simulink model "mvdc_mpc"  (R2018b)
settings: configuration reference "Active" (kept outside this file)
undefined symbols (not defined in the file): A_VehicleReference_m2, acc_control_learning, ax_lim_mps2, ay_lim_mps2, DiscIntNeverNeededParam, drag_coefficient, l_front_m, l_rear_m, LatAcc_cov_debug, LatAcc_FFweights, LatAcc_mean_debug, LongAcc_FFweights, P_VDC_axFFModelLearningEnable, P_VDC_axFFModelLearningRate, P_VDC_axFFModelLearningReg, P_VDC_ayFFModelLearningEnable, P_VDC_ayFFModelLearningRate, P_VDC_ayFFModelLearningReg, P_VDC_Dist_ax_perc, P_VDC_Dist_ay_perc, P_VDC_EnableNumLatErrorDer_b, P_VDC_EnableTubeMPC, P_VDC_EnableUncertaintyLearning, P_VDC_EnableYawRateAccRepl, P_VDC_LatAcc_BetaGain, P_VDC_LatAcc_EnableForesightFF, P_VDC_LatAcc_FF_Ts, P_VDC_LatAcc_Steering_Ts, P_VDC_LatAcc_UndersteerComp_Ts, P_VDC_LatAcc_VehicleDynamics_Ts, P_VDC_LatAccKi, P_VDC_LatAccKi_Lim_perc, P_VDC_LatAccKp_ay, P_VDC_LatAccKp_Delta, P_VDC_LatErrorDer_Ts_s, P_VDC_LongAcc_EnableForesightFF, P_VDC_LongAcc_FB_Ts, P_VDC_LongAcc_FF_Ts, P_VDC_LongAcc_LimFb_N, P_VDC_LongAccKp, P_VDC_MaxTightening, P_VDC_MinVelSlipCalc_mps, P_VDC_PositiveAxLimScale, P_VDC_StabilizerRearSideSlip_rad, P_VDC_SteeringOvalComp_rad, P_VDC_SteeringSteadyStateUndersteerComp_rad, P_VDC_UncertaintyLearningGain, P_VDC_UncertaintyLearningSamples, P_VDC_UncertaintyTarget_perc, P_VDC_VirtualController, Pos, roh_air, sys, tS, tSSlow, TUMHealthStatus, v_mps, vehiclemass_kg
libraries: simulink x31
(part 1 of 2)
settings Model: DataDictionary=mvdc_mpc.sldd  PauseTimes=19.88  Creator=wischnewski  LastModifiedBy=ge34qer

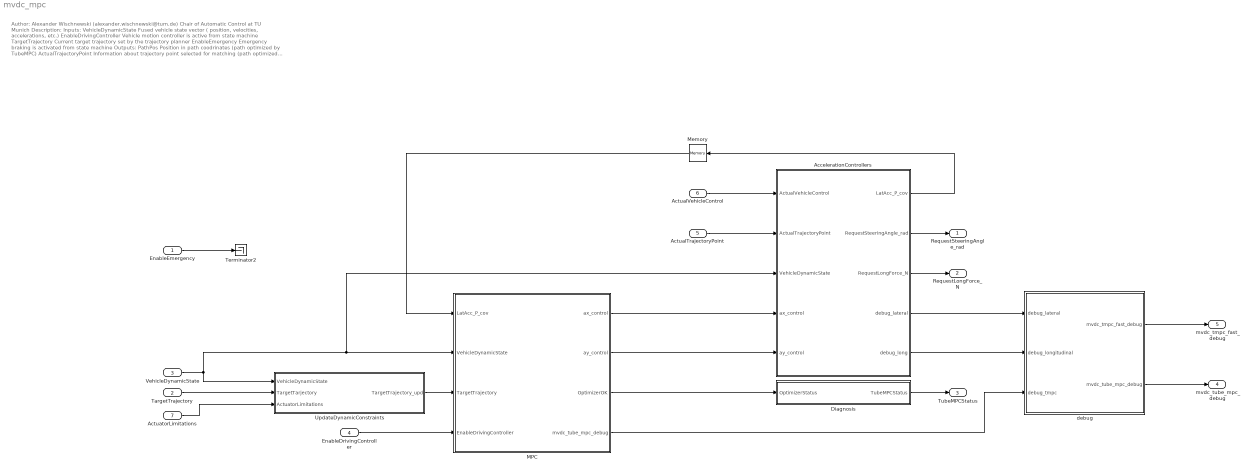
== system mvdc_mpc ==
  note: Author: Alexander Wischnewski (alexander.wischnewski@tum.de)
      | Chair of Automatic Control at TU Munich
      |
      | Description:
      |
      | Inputs:
      | VehicleDynamicState Fused vehicle state vector ( position, velocities, accelerations, etc.)
      | EnableDrivingController Vehicle motion controller is active from state machine
      | TargetTrajectory Current target trajectory set by the trajectory planner
      | EnableEmergency Emergency braking is activated from state machine
      |
      | Outputs:
      | PathPos Position in path coodrinates (path optimized by TubeMPC)
      | ActualTrajectoryPoint Information about trajectory point selected for matching (path optimized by TubeMPC)
      | OptimizedTrajectory Trajectory optimized by TubeMPC
      | TubeMPCStatus Status of TubeMPC controller
  EnableEmergency : Inport  OutDataTypeStr=boolean
  TargetTrajectory : Inport  Port=2  OutDataTypeStr=Bus: Trajectory  SampleTime=tS  BusOutputAsStruct=on
  VehicleDynamicState : Inport  Port=3  OutDataTypeStr=Bus: VehicleDynamicState  SampleTime=tS
  EnableDrivingController : Inport  Port=4  OutDataTypeStr=boolean  SampleTime=tS
  ActualTrajectoryPoint : Inport  Port=5  OutDataTypeStr=Bus: TrajectoryPoint  PortDimensions=1  BusOutputAsStruct=on
  ActualVehicleControl : Inport  Port=6  OutDataTypeStr=Bus: VehicleControl
  ActuatorLimitations : Inport  Port=7  OutDataTypeStr=Bus: ActuatorLimitations  BusOutputAsStruct=on
  AccelerationControllers : Subsystem
  Diagnosis : Subsystem
  MPC : Subsystem
  Memory : Memory
  Terminator2 : Terminator
  UpdateDynamicConstraints : Subsystem
  debug : Subsystem
  RequestSteeringAngle_rad : Outport  SampleTime=tS
  RequestLongForce_N : Outport  Port=2  SampleTime=tS
  TubeMPCStatus : Outport  Port=3  OutDataTypeStr=Enum: TUMHealthStatus  SampleTime=tS
  mvdc_tube_mpc_debug : Outport  Port=4  OutDataTypeStr=Bus: mvdc_tube_mpc_debug  SampleTime=tS
  mvdc_tmpc_fast_debug : Outport  Port=5  OutDataTypeStr=Bus: mvdc_tmpc_fast_debug  SampleTime=tS
  wires:
  UpdateDynamicConstraints/1(TargetTrajectory_upd) -> MPC/3(TargetTrajectory)
  VehicleDynamicState/1 -> MPC/2(VehicleDynamicState), AccelerationControllers/3(VehicleDynamicState), UpdateDynamicConstraints/1(VehicleDynamicState)
  Diagnosis/1(TubeMPCStatus) -> TubeMPCStatus/1
  MPC/3(OptimizerOK) -> Diagnosis/1(OptimizerStatus)
  EnableEmergency/1 -> Terminator2/1
  AccelerationControllers/2(RequestSteeringAngle_rad) -> RequestSteeringAngle_rad/1
  AccelerationControllers/3(RequestLongForce_N) -> RequestLongForce_N/1
  MPC/1(ax_control) -> AccelerationControllers/4(ax_control)
  MPC/2(ay_control) -> AccelerationControllers/5(ay_control)
  AccelerationControllers/4(debug_lateral) -> debug/1(debug_lateral)
  AccelerationControllers/5(debug_long) -> debug/2(debug_longitudinal)
  MPC/4(mvdc_tube_mpc_debug) -> debug/3(debug_tmpc)
  ActualVehicleControl/1 -> AccelerationControllers/1(ActualVehicleControl)
  debug/1(mvdc_tmpc_fast_debug) -> mvdc_tmpc_fast_debug/1
  debug/2(mvdc_tube_mpc_debug) -> mvdc_tube_mpc_debug/1
  ActualTrajectoryPoint/1 -> AccelerationControllers/2(ActualTrajectoryPoint)
  ActuatorLimitations/1 -> UpdateDynamicConstraints/3(ActuatorLimitations)
  TargetTrajectory/1 -> UpdateDynamicConstraints/2(TargetTarjectory)
  Memory/1 -> MPC/1(LatAcc_P_cov)
  AccelerationControllers/1(LatAcc_P_cov) -> Memory/1
  EnableDrivingController/1 -> MPC/4(EnableDrivingController)

== system mvdc_mpc/AccelerationControllers ==
  note: These controllers add small correction signal to the requested steering angle
      | and longitudinal force to counteract small uncertainties in the request characteristics.
      |
      | They do not interfer with the constraint satisfaction generated by the TMPC controller
      | as it is assumed that the measured accelerations are correct and therefore the controller
      | only compensates errors in the request characteristic.
  ActualVehicleControl : Inport
  ActualTrajectoryPoint : Inport  Port=2  OutDataTypeStr=Bus: TrajectoryPoint  PortDimensions=1  BusOutputAsStruct=on
  VehicleDynamicState : Inport  Port=3
  ax_control : Inport  Port=4
  ay_control : Inport  Port=5
  LateralController : Subsystem
  LongitudinalController : Subsystem
  Terminator : Terminator
  LatAcc_P_cov : Outport
  RequestSteeringAngle_rad : Outport  Port=2  SampleTime=tS
  RequestLongForce_N : Outport  Port=3  SampleTime=tS
  debug_lateral : Outport  Port=4
  debug_long : Outport  Port=5
  wires:
  VehicleDynamicState/1 -> LongitudinalController/2(VehicleDynamicState), LateralController/1(VehicleDynamicState)
  ay_control/1 -> LateralController/2(Target_ay_mps2)
  LateralController/1(RequestSteeringAngle_rad) -> RequestSteeringAngle_rad/1
  ax_control/1 -> LongitudinalController/3(Target_ax_mps2)
  LongitudinalController/1(RequestLongForce_N) -> RequestLongForce_N/1
  LateralController/2(debug) -> debug_lateral/1
  LongitudinalController/2(debug) -> debug_long/1
  ActualVehicleControl/1 -> Terminator/1
  ActualTrajectoryPoint/1 -> LateralController/3(ActualTrajectoryPoint)
  LateralController/3(LatAcc_P_cov) -> LatAcc_P_cov/1
  LateralController/4(StabilizerActive) -> LongitudinalController/1(StabilizerActive)

== system mvdc_mpc/Diagnosis ==
  OptimizerStatus : Inport
  Constant : Constant  Value=TUMHealthStatus.OK
  Constant1 : Constant  Value=TUMHealthStatus.ERROR
  Switch : Switch  Criteria=u2 > Threshold
  TubeMPCStatus : Outport
  wires:
  Switch/1 -> TubeMPCStatus/1
  OptimizerStatus/1 -> Switch/2
  Constant/1 -> Switch/1
  Constant1/1 -> Switch/3

== system mvdc_mpc/MPC ==
  LatAcc_P_cov : Inport
  VehicleDynamicState : Inport  Port=2  OutDataTypeStr=Bus: VehicleDynamicState
  TargetTrajectory : Inport  Port=3  OutDataTypeStr=Bus: Trajectory
  EnableDrivingController : Inport  Port=4  OutDataTypeStr=boolean  SampleTime=tS
  Bus Selector : BusSelector  OutputSignals=ax_pred_mps2,ay_pred_mps2
  Debug : Subsystem
  DelayCompensation : Subsystem
  DisturbanceEstimation : Subsystem
  Memory : Memory  InheritSampleTime=on
  Memory1 : Memory  InheritSampleTime=on
  TubeMPC : Subsystem  TreatAsAtomicUnit=on
  VehicleReadyForTMPC : Subsystem
  ax_control : Outport
  ay_control : Outport  Port=2
  OptimizerOK : Outport  Port=3  OutDataTypeStr=boolean
  mvdc_tube_mpc_debug : Outport  Port=4  OutDataTypeStr=Bus: mvdc_tube_mpc_debug
  wires:
  TargetTrajectory/1 -> VehicleReadyForTMPC/2(TargetTrajectory), TubeMPC/5(TargetTrajectory), Debug/9(TargetTrajectory)
  VehicleDynamicState/1 -> DelayCompensation/1(VehicleDynamicState), DisturbanceEstimation/3(VehicleDynamicState), VehicleReadyForTMPC/1(VehicleDynamicState)
  Debug/1(mvdc_tube_mpc_debug) -> mvdc_tube_mpc_debug/1
  TubeMPC/3(solver_details) -> Debug/4(solver_details)
  TubeMPC/2(exitflags) -> Debug/3(exit_flags)
  TubeMPC/5(MiscDebug) -> Debug/6(MiscDebug)
  TubeMPC/4(ResampledTargetTrajectory) -> Debug/5(ResampledTargetTrajectory)
  TubeMPC/1(OptimizerOK) -> OptimizerOK/1
  TubeMPC/7(Linearization) -> Debug/8(LinearizationDebug)
  DelayCompensation/1(VehicleDynamicStateUpdated) -> TubeMPC/1(VehicleDynamicState), Debug/2(VehicleDynamicState)
  Memory/1 -> DisturbanceEstimation/1(ax_control_mps2)
  Memory1/1 -> DisturbanceEstimation/2(ay_control_mps2)
  DisturbanceEstimation/2(M_tilde) -> TubeMPC/2(M_tilde)
  DisturbanceEstimation/1(debug) -> Debug/1(debug_distLearning)
  TubeMPC/6(Prediction) -> Bus Selector/1, Debug/7(PredictionDebug)
  Bus Selector/1 -> Memory/1, ax_control/1  "<ax_pred_mps2>"
  Bus Selector/2 -> ay_control/1, Memory1/1  "<ay_pred_mps2>"
  LatAcc_P_cov/1 -> TubeMPC/4(LatAcc_P_cov)
  VehicleReadyForTMPC/1(VehicleReadyForTMPC) -> DisturbanceEstimation/4(VehicleReadyForTMPC), TubeMPC/Enable
  EnableDrivingController/1 -> VehicleReadyForTMPC/3(EnableDrivingController)
  VehicleReadyForTMPC/2(StartTMPC) -> TubeMPC/3(StartTMPC)

== system mvdc_mpc/UpdateDynamicConstraints ==
  note: reduce the max. long acceleration at standstill
      | to prevent excessive wheelspin at the start.
  note: calculates the maximum possible lateral acceleration
      | at low speeds and checks whether the steering angle
      | limits the achievable lateral acceleration.
  VehicleDynamicState : Inport  OutDataTypeStr=Bus: VehicleDynamicState  SampleTime=tS
  TargetTarjectory : Inport  Port=2
  ActuatorLimitations : Inport  Port=3  OutDataTypeStr=Bus: ActuatorLimitations  BusOutputAsStruct=on
  Bus Assignment : BusAssignment  AssignedSignals=ax_lim_mps2,ay_lim_mps2
  Bus Selector : BusSelector  OutputSignals=SteeringAngleMax_rad
  Bus Selector1 : BusSelector  OutputSignals=v_mps
  Bus Selector2 : BusSelector  OutputSignals=ay_lim_mps2
  Bus Selector3 : BusSelector  OutputSignals=ax_lim_mps2
  Constant : Constant  Value=P_VDC_MinVelSlipCalc_mps
  Gain : Gain  Gain=1/(l_front_m+l_rear_m)
  Gain1 : Gain  Gain=1/3
  Min : MinMax  Inputs=2
  Min1 : MinMax  Function=max  Inputs=2
  Multiply : Product
  Square : Math  Operator=square  SaturateOnIntegerOverflow=on
  Switch : Switch  Criteria=u2 > Threshold  Threshold=P_VDC_MinVelSlipCalc_mps
  TargetTrajectory_upd : Outport
  wires:
  ActuatorLimitations/1 -> Bus Selector/1
  Bus Selector/1 -> Gain/1  "<SteeringAngleMax_rad>"
  VehicleDynamicState/1 -> Bus Selector1/1
  Square/1 -> Multiply/2
  Gain/1 -> Multiply/1
  Bus Selector2/1 -> Min/1  "<ay_lim_mps2>"
  Min/1 -> Bus Assignment/3
  Bus Assignment/1 -> TargetTrajectory_upd/1
  Bus Selector1/1 -> Switch/2, Min1/1  "<v_mps>"
  Constant/1 -> Min1/2
  Min1/1 -> Square/1
  Multiply/1 -> Min/2
  TargetTarjectory/1 -> Bus Assignment/1, Bus Selector2/1, Bus Selector3/1
  Switch/1 -> Bus Assignment/2
  Bus Selector3/1 -> Gain1/1, Switch/1  "<ax_lim_mps2>"
  Gain1/1 -> Switch/3

== system mvdc_mpc/debug ==
  note: the tmpc_cnt enables sync between different logging rates
  debug_lateral : Inport
  debug_longitudinal : Inport  Port=2
  debug_tmpc : Inport  Port=3
  Bus Assignment : BusAssignment  AssignedSignals=LongAcc_FFweights,LatAcc_FFweights,LatAcc_mean_debug,LatAcc_cov_debug
  Bus Creator : BusCreator  Inputs=39
  Bus Selector : BusSelector  OutputSignals=LatAcc_bank_mps2,LatAcc_FB_Dist_rad,LatAcc_FB_ay_rad,LatAcc_FB_Delta_rad,LatAcc_FFss_rad,LatAcc_FFdyn_rad,LatAcc_Control_rad,LatAcc_Target_mps2,LatAcc_VirtualAccTarget_mps2,LatAcc_VirtualSteeringTarget_rad,LatAcc_FFLearned_rad,LatAcc_DiffToNeutralSteer_rad,LatAcc_FBStabilizer_rad
  Bus Selector1 : BusSelector  OutputSignals=LongAcc_FB_N,LongAcc_FFax_N,LongAcc_FFdist_N,LongAcc_Control_N,LongAcc_Target_mps2,LongAcc_TargetFF_mps2,LongAcc_FFLearned_N
  Bus Selector2 : BusSelector  OutputSignals=cost_values,solver_iteration,solver_state,solver_runTime_s,solver_pri_res,solver_dua_res,tmpc_cnt,TireUtilizationTarget,ax_LearnedBound_mps2,ax_DataCoverage_perc,ax_Uncertainty_mps2,ay_LearnedBound_mps2,ay_DataCoverage_perc,ay_Uncertainty_mps2,dot_d_analytical_mps,dot_d_numerical_mps
  Bus Selector3 : BusSelector  OutputSignals=LatAcc_FFweights,LatAcc_mean_debug,LatAcc_cov_debug
  Bus Selector4 : BusSelector  OutputSignals=LongAcc_FFweights
  Demux : Demux
  Signal Copy{2..5} (4 alike) : SignalConversion  OverrideOpt=off
  mvdc_tmpc_fast_debug : Outport
  mvdc_tube_mpc_debug : Outport  Port=2  OutDataTypeStr=Bus: mvdc_tube_mpc_debug  SampleTime=tS
  wires:
  debug_longitudinal/1 -> Bus Selector4/1, Bus Selector1/1
  Bus Selector1/2 -> Bus Creator/15  "<LongAcc_FFax_N>"
  Bus Selector/5 -> Bus Creator/5  "<LatAcc_FFss_rad>"
  Bus Selector/3 -> Bus Creator/3  "<LatAcc_FB_ay_rad>"
  Bus Selector/7 -> Bus Creator/7  "<LatAcc_Control_rad>"
  Bus Selector1/3 -> Bus Creator/16  "<LongAcc_FFdist_N>"
  Bus Selector1/4 -> Bus Creator/17  "<LongAcc_Control_N>"
  debug_lateral/1 -> Bus Selector3/1, Bus Selector/1
  Bus Selector2/7 -> Bus Creator/30  "<tmpc_cnt>"
  Bus Selector/8 -> Bus Creator/8  "<LatAcc_Target_mps2>"
  Bus Selector1/5 -> Bus Creator/18  "<LongAcc_Target_mps2>"
  Bus Selector2/2 -> Bus Creator/25  "<solver_iteration>"
  Bus Selector2/1 -> Demux/1  "<cost_values>"
  Demux/1 -> Signal Copy2/1
  Demux/2 -> Signal Copy3/1
  Signal Copy3/1 -> Bus Creator/22  "input_cost"
  Demux/3 -> Signal Copy4/1
  Signal Copy4/1 -> Bus Creator/23  "reg_cost"
  Demux/4 -> Signal Copy5/1
  Signal Copy5/1 -> Bus Creator/24  "slack_cost"
  Bus Selector2/4 -> Bus Creator/27  "<solver_runTime_s>"
  Bus Selector2/5 -> Bus Creator/28  "<solver_pri_res>"
  Bus Selector2/6 -> Bus Creator/29  "<solver_dua_res>"
  Bus Creator/1 -> mvdc_tmpc_fast_debug/1
  Bus Selector/11 -> Bus Creator/11  "<LatAcc_FFLearned_rad>"
  Bus Selector1/1 -> Bus Creator/14  "<LongAcc_FB_N>"
  Signal Copy2/1 -> Bus Creator/21  "state_cost"
  Bus Selector2/3 -> Bus Creator/26  "<solver_state>"
  Bus Selector2/8 -> Bus Creator/31  "<TireUtilizationTarget>"
  Bus Selector2/9 -> Bus Creator/32  "<ax_LearnedBound_mps2>"
  Bus Selector2/10 -> Bus Creator/33  "<ax_DataCoverage_perc>"
  Bus Selector2/12 -> Bus Creator/35  "<ay_LearnedBound_mps2>"
  Bus Selector2/13 -> Bus Creator/36  "<ay_DataCoverage_perc>"
  Bus Selector2/11 -> Bus Creator/34  "<ax_Uncertainty_mps2>"
  Bus Selector2/14 -> Bus Creator/37  "<ay_Uncertainty_mps2>"
  Bus Selector1/7 -> Bus Creator/20  "<LongAcc_FFLearned_N>"
  debug_tmpc/1 -> Bus Assignment/1, Bus Selector2/1
  Bus Assignment/1 -> mvdc_tube_mpc_debug/1
  Bus Selector3/1 -> Bus Assignment/3  "<LatAcc_FFweights>"
  Bus Selector4/1 -> Bus Assignment/2  "<LongAcc_FFweights>"
  Bus Selector/9 -> Bus Creator/9  "<LatAcc_VirtualAccTarget_mps2>"
  Bus Selector1/6 -> Bus Creator/19  "<LongAcc_TargetFF_mps2>"
  Bus Selector/6 -> Bus Creator/6  "<LatAcc_FFdyn_rad>"
  Bus Selector/1 -> Bus Creator/1  "<LatAcc_bank_mps2>"
  Bus Selector/4 -> Bus Creator/4  "<LatAcc_FB_Delta_rad>"
  Bus Selector/10 -> Bus Creator/10  "<LatAcc_VirtualSteeringTarget_rad>"
  Bus Selector/2 -> Bus Creator/2  "<LatAcc_FB_Dist_rad>"
  Bus Selector3/2 -> Bus Assignment/4  "<LatAcc_mean_debug>"
  Bus Selector3/3 -> Bus Assignment/5  "<LatAcc_cov_debug>"
  Bus Selector/12 -> Bus Creator/12  "<LatAcc_DiffToNeutralSteer_rad>"
  Bus Selector/13 -> Bus Creator/13  "<LatAcc_FBStabilizer_rad>"
  Bus Selector2/15 -> Bus Creator/38  "<dot_d_analytical_mps>"
  Bus Selector2/16 -> Bus Creator/39  "<dot_d_numerical_mps>"

== system mvdc_mpc/AccelerationControllers/LateralController ==
  note: used to disable throttle in case
      | stabilizer kicks in
  VehicleDynamicState : Inport
  Target_ay_mps2 : Inport  Port=2
  ActualTrajectoryPoint : Inport  Port=3  OutDataTypeStr=Bus: TrajectoryPoint  PortDimensions=1  BusOutputAsStruct=on
  Abs : Abs
  Add : Sum  Inputs=+++++++
  Add1 : Sum  Inputs=++++++
  Bus Creator : BusCreator  Inputs=16
  Bus Selector : BusSelector  OutputSignals=ay_lim_mps2
  Bus Selector1 : BusSelector  OutputSignals=valid_IMU_b,alphaRL_rad,alphaRR_rad,DeltaWheel_rad,dPsi_radps,ay_mps2,v_mps
  Compare To Constant : simulink/Logic and Bit Operations/Compare To Constant  relop=>  const=0  OutDataTypeStr=boolean
  Constant : Constant  Value=0
  Feedback : Subsystem
  Feedforward_InverseModel : Subsystem
  Feedforward_Learning : Subsystem
  Selector : Selector  InputPortWidth=sys.N_hor+1  IndexOptions=Index vector (dialog)  Indices=1  OutputSizes=1
  Unit Delay1 : UnitDelay  SampleTime=-1
  RequestSteeringAngle_rad : Outport
  debug : Outport  Port=2
  LatAcc_P_cov : Outport  Port=3
  StabilizerActive : Outport  Port=4
  wires:
  Target_ay_mps2/1 -> Feedforward_InverseModel/2(LatAcc_Target_mps2), Selector/1
  VehicleDynamicState/1 -> Bus Selector1/1
  Add/1 -> Bus Creator/11, RequestSteeringAngle_rad/1  "LatAcc_Control_rad"
  Bus Creator/1 -> debug/1
  Feedforward_InverseModel/4(LatAcc_FFss_rad) -> Bus Creator/9, Add/4  "LatAcc_FFss_rad"
  Feedback/3(LatAcc_FB_ay_rad) -> Add1/2, Add/2, Bus Creator/3  "LatAcc_FB_ay_rad"
  Bus Selector1/6 -> Feedforward_Learning/2(ay_mps2), Feedback/6(ay_mps2)  "<ay_mps2>"
  Bus Selector1/7 -> Feedforward_Learning/1(v_mps), Feedforward_InverseModel/3(v_mps), Feedback/7(v_mps)  "<v_mps>"
  Selector/1 -> Bus Creator/7  "LatAcc_Target_mps2"
  Feedforward_InverseModel/1(LatAcc_VirtualAccTarget_mps2) -> Feedback/9(LatAcc_VirtualTarget_mps2), Bus Creator/5  "LatAcc_VirtualAccTarget_mps2"
  Feedforward_InverseModel/6(LatAcc_FFLearned_rad) -> Bus Creator/12, Add1/6, Add/6  "LatAcc_FFLearned_rad"
  Feedforward_Learning/1(LatAcc_FFweights) -> Bus Creator/14, Feedforward_InverseModel/4(LatAcc_FFweights)  "LatAcc_FFweights"
  Bus Selector1/5 -> Feedback/5(dPsi_radps)  "<dPsi_radps>"
  Feedforward_InverseModel/5(LatAcc_FFdyn_rad) -> Bus Creator/10, Add1/5, Add/5  "LatAcc_FFdyn_rad"
  Feedforward_InverseModel/3(SideSlipCompensation_YawRate_radps) -> Feedback/11(SideSlipCompensation_YawRate_radps)
  Unit Delay1/1 -> Bus Creator/13, Feedforward_Learning/3(DiffToNeutralSteer_rad)  "LatAcc_DiffToNeutralSteer_rad"
  Add1/1 -> Unit Delay1/1
  ActualTrajectoryPoint/1 -> Bus Selector/1, Feedforward_InverseModel/5(ActualTrajectoryPoint)
  Constant/1 -> Bus Creator/8  "LatAcc_bank_mps2"
  Feedforward_InverseModel/2(LatAcc_VirtualSteeringTarget_rad) -> Bus Creator/6, Feedback/10(LatAcc_VirtualSteeringTarget_rad)  "LatAcc_VirtualSteeringTarget_rad"
  Bus Selector1/4 -> Feedback/4(DeltaWheel_rad)  "<DeltaWheel_rad>"
  Feedback/4(LatAcc_FB_Delta_rad) -> Add1/1, Add/3, Bus Creator/4  "LatAcc_FB_Delta_rad"
  Feedback/2(LatAcc_FB_Dist_rad) -> Bus Creator/2, Add1/3, Add/1  "LatAcc_FB_Dist_rad"
  Feedforward_Learning/2(LatAcc_P_cov) -> LatAcc_P_cov/1
  Feedforward_Learning/3(LatAcc_mean_debug) -> Bus Creator/15  "LatAcc_mean_debug"
  Feedforward_Learning/4(LatAcc_cov_debug) -> Bus Creator/16  "LatAcc_cov_debug"
  Feedback/1(LatAcc_FBStabilizer_rad) -> Add1/4, Add/7, Bus Creator/1, Abs/1  "LatAcc_FBStabilizer_rad"
  Bus Selector1/2 -> Feedback/2(alphaRL_rad)  "<alphaRL_rad>"
  Bus Selector/1 -> Feedback/8(LatAcc_Limit_mps2)  "<ay_lim_mps2>"
  Bus Selector1/3 -> Feedback/3(alphaRR_rad)  "<alphaRR_rad>"
  Abs/1 -> Compare To Constant/1
  Compare To Constant/1 -> StabilizerActive/1
  Bus Selector1/1 -> Feedforward_InverseModel/1(valid_IMU_b), Feedback/1(valid_IMU_b)  "<valid_IMU_b>"

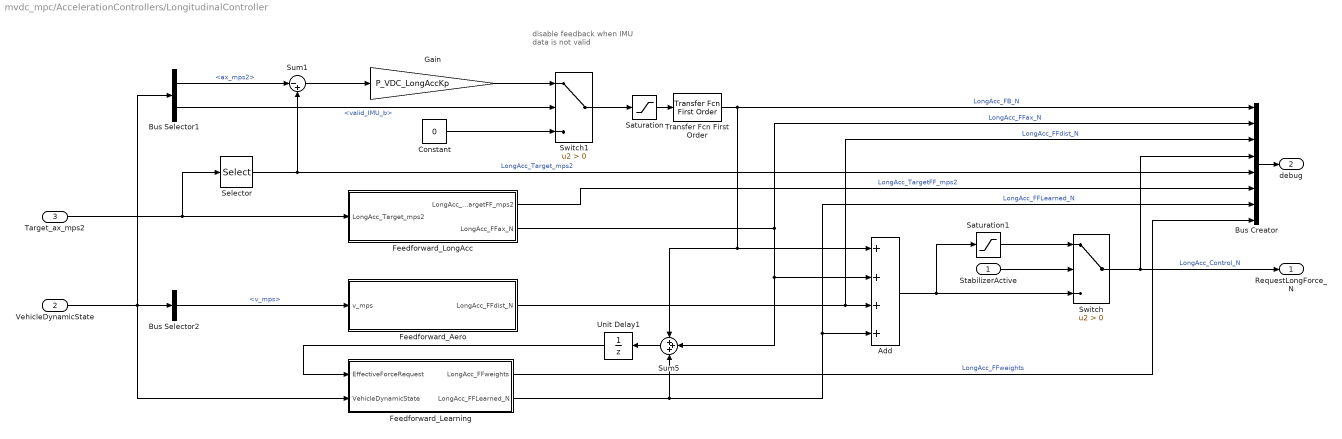
== system mvdc_mpc/AccelerationControllers/LongitudinalController ==
  note: disable feedback when
      | IMU data is not valid
  StabilizerActive : Inport
  VehicleDynamicState : Inport  Port=2
  Target_ax_mps2 : Inport  Port=3
  Add : Sum  Inputs=++++
  Bus Creator : BusCreator  Inputs=8
  Bus Selector1 : BusSelector  OutputSignals=ax_mps2,valid_IMU_b
  Bus Selector2 : BusSelector  OutputSignals=v_mps
  Constant : Constant  Value=0
  Feedforward_Aero : Subsystem
  Feedforward_Learning : Subsystem
  Feedforward_LongAcc : Subsystem
  Gain : Gain  Gain=P_VDC_LongAccKp
  Saturation : Saturate  UpperLimit=P_VDC_LongAcc_LimFb_N  LowerLimit=-P_VDC_LongAcc_LimFb_N
  Saturation1 : Saturate  UpperLimit=0  LowerLimit=-inf
  Selector : Selector  InputPortWidth=sys.N_hor+1  IndexOptions=Index vector (dialog)  Indices=[1]  OutputSizes=1
  Sum1 : Sum  Inputs=|-+
  Sum5 : Sum  Inputs=+++
  Switch : Switch  Criteria=u2 > Threshold
  Switch1 : Switch  Criteria=u2 > Threshold
  Transfer Fcn First Order : simulink/Discrete/Transfer Fcn First Order  PoleZ=exp(-tS/P_VDC_LongAcc_FB_Ts)  ICPrevOutput=0.0  DoSatur=off
      settings: SourceProductName=Simulink
  Unit Delay1 : UnitDelay  SampleTime=-1
  RequestLongForce_N : Outport
  debug : Outport  Port=2
  wires:
  Switch/1 -> Bus Creator/4, RequestLongForce_N/1  "LongAcc_Control_N"
  Bus Selector2/1 -> Feedforward_Aero/1(v_mps)  "<v_mps>"
  VehicleDynamicState/1 -> Feedforward_Learning/2(VehicleDynamicState), Bus Selector1/1, Bus Selector2/1
  Bus Selector1/1 -> Sum1/1  "<ax_mps2>"
  Sum1/1 -> Gain/1
  Bus Creator/1 -> debug/1
  Target_ax_mps2/1 -> Selector/1, Feedforward_LongAcc/1(LongAcc_Target_mps2)
  Feedforward_Learning/2(LongAcc_FFLearned_N) -> Bus Creator/7, Add/4, Sum5/3  "LongAcc_FFLearned_N"
  Feedforward_LongAcc/2(LongAcc_FFax_N) -> Sum5/2, Add/2, Bus Creator/2  "LongAcc_FFax_N"
  Feedforward_Aero/1(LongAcc_FFdist_N) -> Bus Creator/3, Add/3  "LongAcc_FFdist_N"
  Selector/1 -> Sum1/2, Bus Creator/5  "LongAcc_Target_mps2"
  Feedforward_LongAcc/1(LongAcc_TargetFF_mps2) -> Bus Creator/6  "LongAcc_TargetFF_mps2"
  Sum5/1 -> Unit Delay1/1
  Feedforward_Learning/1(LongAcc_FFweights) -> Bus Creator/8  "LongAcc_FFweights"
  Unit Delay1/1 -> Feedforward_Learning/1(EffectiveForceRequest)
  Transfer Fcn First Order/1 -> Bus Creator/1, Sum5/1, Add/1  "LongAcc_FB_N"
  Saturation/1 -> Transfer Fcn First Order/1
  Add/1 -> Switch/3, Saturation1/1
  StabilizerActive/1 -> Switch/2
  Saturation1/1 -> Switch/1
  Gain/1 -> Switch1/1
  Switch1/1 -> Saturation/1
  Bus Selector1/2 -> Switch1/2  "<valid_IMU_b>"
  Constant/1 -> Switch1/3

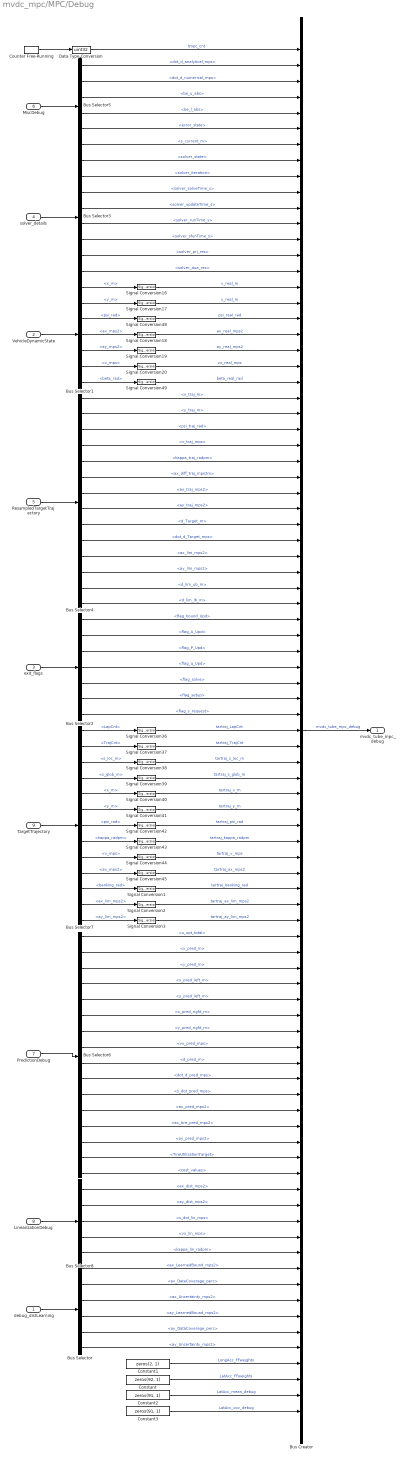
== system mvdc_mpc/MPC/Debug ==
  debug_distLearning : Inport
  VehicleDynamicState : Inport  Port=2
  exit_flags : Inport  Port=3
  solver_details : Inport  Port=4
  ResampledTargetTrajectory : Inport  Port=5
  MiscDebug : Inport  Port=6
  PredictionDebug : Inport  Port=7
  LinearizationDebug : Inport  Port=8
  TargetTrajectory : Inport  Port=9
  Bus Creator : BusCreator  Inputs=87
  Bus Selector : BusSelector  OutputSignals=ax_LearnedBound_mps2,ax_DataCoverage_perc,ax_Uncertainty_mps2,ay_LearnedBound_mps2,ay_DataCoverage_perc,ay_Uncertainty_mps2
  Bus Selector1 : BusSelector  OutputSignals=Pos.x_m,Pos.y_m,Pos.psi_rad,ax_mps2,ay_mps2,v_mps,beta_rad
  Bus Selector2 : BusSelector  OutputSignals=flag_bound_Upd,flag_A_Upd,flag_P_Upd,flag_q_Upd,flag_solve,flag_setup,flag_s_request
  Bus Selector3 : BusSelector  OutputSignals=solver_state,solver_iteration,solver_solveTime_s,solver_updateTime_s,solver_runTime_s,solver_sfunTime_s,solver_pri_res,solver_dua_res
  Bus Selector4 : BusSelector  OutputSignals=x_traj_m,y_traj_m,psi_traj_rad,v_traj_mps,kappa_traj_radpm,ax_diff_traj_mps2m,ax_traj_mps2,ay_traj_mps2,d_Target_m,dot_d_Target_mps,ax_lim_mps2,ay_lim_mps2,d_lim_ub_m,d_lim_lb_m
  Bus Selector5 : BusSelector  OutputSignals=dot_d_analytical_mps,dot_d_numerical_mps,be_u_abs,be_l_abs,error_state,s_current_m
  Bus Selector6 : BusSelector  OutputSignals=u_opt_total,x_pred_m,y_pred_m,x_pred_left_m,y_pred_left_m,x_pred_right_m,y_pred_right_m,vx_pred_mps,d_pred_m,dot_d_pred_mps,s_dot_pred_mps,ax_pred_mps2,ax_tire_pred_mps2,ay_pred_mps2,TireUtilizationTarget,cost_values
  Bus Selector7 : BusSelector  OutputSignals=LapCnt,TrajCnt,s_loc_m,s_glob_m,x_m,y_m,psi_rad,kappa_radpm,v_mps,ax_mps2,banking_rad,ax_lim_mps2,ay_lim_mps2
  Bus Selector8 : BusSelector  OutputSignals=ax_dist_mps2,ay_dist_mps2,s_dot_lin_mps,vx_lin_mps,kappa_lin_radpm
  Constant : Constant  Value=zeros(92, 1)
  Constant1 : Constant  Value=zeros(2, 1)
  Constant2 : Constant  Value=zeros(91, 1)
  Constant3 : Constant  Value=zeros(91, 1)
  Counter Free-Running : simulink/Sources/Counter Free-Running  NumBits=32  tsamp=-1
  Data Type Conversion : DataTypeConversion  OutDataTypeStr=uint32
  Signal Conversion{1..3,16..20,36..45,48..49} (20 alike) : SignalConversion  OverrideOpt=off
  mvdc_tube_mpc_debug : Outport
  wires:
  Signal Conversion17/1 -> Bus Creator/17  "y_real_m"
  Signal Conversion19/1 -> Bus Creator/20  "ay_real_mps2"
  Signal Conversion16/1 -> Bus Creator/16  "x_real_m"
  Bus Selector1/4 -> Signal Conversion18/1  "<ax_mps2>"
  Signal Conversion20/1 -> Bus Creator/21  "vx_real_mps"
  Bus Selector1/6 -> Signal Conversion20/1  "<v_mps>"
  Bus Creator/1 -> mvdc_tube_mpc_debug/1  "mvdc_tube_mpc_debug"
  Bus Selector1/2 -> Signal Conversion17/1  "<y_m>"
  Bus Selector1/5 -> Signal Conversion19/1  "<ay_mps2>"
  Bus Selector1/1 -> Signal Conversion16/1  "<x_m>"
  Signal Conversion18/1 -> Bus Creator/19  "ax_real_mps2"
  exit_flags/1 -> Bus Selector2/1
  Bus Selector2/1 -> Bus Creator/37  "<flag_bound_Upd>"
  Bus Selector2/2 -> Bus Creator/38  "<flag_A_Upd>"
  Bus Selector2/3 -> Bus Creator/39  "<flag_P_Upd>"
  Bus Selector2/4 -> Bus Creator/40  "<flag_q_Upd>"
  Bus Selector2/5 -> Bus Creator/41  "<flag_solve>"
  Bus Selector2/6 -> Bus Creator/42  "<flag_setup>"
  solver_details/1 -> Bus Selector3/1
  Bus Selector3/1 -> Bus Creator/8  "<solver_state>"
  Bus Selector3/2 -> Bus Creator/9  "<solver_iteration>"
  Bus Selector3/3 -> Bus Creator/10  "<solver_solveTime_s>"
  Bus Selector3/4 -> Bus Creator/11  "<solver_updateTime_s>"
  Bus Selector3/5 -> Bus Creator/12  "<solver_runTime_s>"
  Bus Selector3/6 -> Bus Creator/13  "<solver_sfunTime_s>"
  ResampledTargetTrajectory/1 -> Bus Selector4/1
  Bus Selector4/1 -> Bus Creator/23  "<x_traj_m>"
  Bus Selector4/2 -> Bus Creator/24  "<y_traj_m>"
  Bus Selector4/3 -> Bus Creator/25  "<psi_traj_rad>"
  Bus Selector4/4 -> Bus Creator/26  "<v_traj_mps>"
  MiscDebug/1 -> Bus Selector5/1
  VehicleDynamicState/1 -> Bus Selector1/1
  Bus Selector2/7 -> Bus Creator/43  "<flag_s_request>"
  TargetTrajectory/1 -> Bus Selector7/1
  Bus Selector7/1 -> Signal Conversion36/1  "<LapCnt>"
  Bus Selector7/2 -> Signal Conversion37/1  "<TrajCnt>"
  Bus Selector7/3 -> Signal Conversion38/1  "<s_loc_m>"
  Bus Selector7/4 -> Signal Conversion39/1  "<s_glob_m>"
  Bus Selector7/5 -> Signal Conversion40/1  "<x_m>"
  Bus Selector7/6 -> Signal Conversion41/1  "<y_m>"
  Bus Selector7/7 -> Signal Conversion42/1  "<psi_rad>"
  Bus Selector7/8 -> Signal Conversion43/1  "<kappa_radpm>"
  Bus Selector7/9 -> Signal Conversion44/1  "<v_mps>"
  Bus Selector7/10 -> Signal Conversion45/1  "<ax_mps2>"
  Signal Conversion36/1 -> Bus Creator/44  "tartraj_LapCnt"
  Signal Conversion37/1 -> Bus Creator/45  "tartraj_TrajCnt"
  Signal Conversion38/1 -> Bus Creator/46  "tartraj_s_loc_m"
  Signal Conversion39/1 -> Bus Creator/47  "tartraj_s_glob_m"
  Signal Conversion40/1 -> Bus Creator/48  "tartraj_x_m"
  Signal Conversion41/1 -> Bus Creator/49  "tartraj_y_m"
  Signal Conversion42/1 -> Bus Creator/50  "tartraj_psi_rad"
  Signal Conversion43/1 -> Bus Creator/51  "tartraj_kappa_radpm"
  Signal Conversion44/1 -> Bus Creator/52  "tartraj_v_mps"
  Signal Conversion45/1 -> Bus Creator/53  "tartraj_ax_mps2"
  LinearizationDebug/1 -> Bus Selector8/1
  Bus Selector1/3 -> Signal Conversion48/1  "<psi_rad>"
  Signal Conversion49/1 -> Bus Creator/22  "beta_real_rad"
  Bus Selector1/7 -> Signal Conversion49/1  "<beta_rad>"
  Signal Conversion48/1 -> Bus Creator/18  "psi_real_rad"
  Bus Selector3/8 -> Bus Creator/15  "<solver_dua_res>"
  Bus Selector3/7 -> Bus Creator/14  "<solver_pri_res>"
  Counter Free-Running/1 -> Data Type Conversion/1
  Data Type Conversion/1 -> Bus Creator/1  "tmpc_cnt"
  Bus Selector4/5 -> Bus Creator/27  "<kappa_traj_radpm>"
  Bus Selector4/6 -> Bus Creator/28  "<ax_diff_traj_mps2m>"
  Bus Selector8/4 -> Bus Creator/76  "<vx_lin_mps>"
  Bus Selector8/3 -> Bus Creator/75  "<s_dot_lin_mps>"
  Bus Selector4/7 -> Bus Creator/29  "<ax_traj_mps2>"
  Bus Selector4/8 -> Bus Creator/30  "<ay_traj_mps2>"
  debug_distLearning/1 -> Bus Selector/1
  Bus Selector/1 -> Bus Creator/78  "<ax_LearnedBound_mps2>"
  Bus Selector/2 -> Bus Creator/79  "<ax_DataCoverage_perc>"
  Bus Selector/4 -> Bus Creator/81  "<ay_LearnedBound_mps2>"
  Bus Selector/5 -> Bus Creator/82  "<ay_DataCoverage_perc>"
  Bus Selector/3 -> Bus Creator/80  "<ax_Uncertainty_mps2>"
  Bus Selector/6 -> Bus Creator/83  "<ay_Uncertainty_mps2>"
  Constant/1 -> Bus Creator/85  "LatAcc_FFweights"
  Constant1/1 -> Bus Creator/84  "LongAcc_FFweights"
  Bus Selector4/9 -> Bus Creator/31  "<d_Target_m>"
  Bus Selector4/10 -> Bus Creator/32  "<dot_d_Target_mps>"
  Bus Selector7/11 -> Signal Conversion1/1  "<banking_rad>"
  Signal Conversion1/1 -> Bus Creator/54  "tartraj_banking_rad"
  Bus Selector7/12 -> Signal Conversion2/1  "<ax_lim_mps2>"
  Signal Conversion2/1 -> Bus Creator/55  "tartraj_ax_lim_mps2"
  Bus Selector7/13 -> Signal Conversion3/1  "<ay_lim_mps2>"
  Signal Conversion3/1 -> Bus Creator/56  "tartraj_ay_lim_mps2"
  Bus Selector8/5 -> Bus Creator/77  "<kappa_lin_radpm>"
  PredictionDebug/1 -> Bus Selector6/1
  Bus Selector6/2 -> Bus Creator/58  "<x_pred_m>"
  Bus Selector6/3 -> Bus Creator/59  "<y_pred_m>"
  Bus Selector6/4 -> Bus Creator/60  "<x_pred_left_m>"
  Bus Selector6/5 -> Bus Creator/61  "<y_pred_left_m>"
  Bus Selector6/6 -> Bus Creator/62  "<x_pred_right_m>"
  Bus Selector6/7 -> Bus Creator/63  "<y_pred_right_m>"
  Bus Selector6/8 -> Bus Creator/64  "<vx_pred_mps>"
  Bus Selector6/9 -> Bus Creator/65  "<d_pred_m>"
  Bus Selector6/10 -> Bus Creator/66  "<dot_d_pred_mps>"
  Bus Selector6/11 -> Bus Creator/67  "<s_dot_pred_mps>"
  Bus Selector6/12 -> Bus Creator/68  "<ax_pred_mps2>"
  Bus Selector6/13 -> Bus Creator/69  "<ax_tire_pred_mps2>"
  Bus Selector6/14 -> Bus Creator/70  "<ay_pred_mps2>"
  Bus Selector6/1 -> Bus Creator/57  "<u_opt_total>"
  Bus Selector6/15 -> Bus Creator/71  "<TireUtilizationTarget>"
  Bus Selector6/16 -> Bus Creator/72  "<cost_values>"
  Bus Selector8/1 -> Bus Creator/73  "<ax_dist_mps2>"
  Bus Selector8/2 -> Bus Creator/74  "<ay_dist_mps2>"
  Bus Selector5/3 -> Bus Creator/4  "<be_u_abs>"
  Bus Selector5/4 -> Bus Creator/5  "<be_l_abs>"
  Bus Selector4/11 -> Bus Creator/33  "<ax_lim_mps2>"
  Bus Selector4/12 -> Bus Creator/34  "<ay_lim_mps2>"
  Bus Selector4/13 -> Bus Creator/35  "<d_lim_ub_m>"
  Bus Selector4/14 -> Bus Creator/36  "<d_lim_lb_m>"
  Bus Selector5/5 -> Bus Creator/6  "<error_state>"
  Bus Selector5/6 -> Bus Creator/7  "<s_current_m>"
  Constant2/1 -> Bus Creator/86  "LatAcc_mean_debug"
  Constant3/1 -> Bus Creator/87  "LatAcc_cov_debug"
  Bus Selector5/1 -> Bus Creator/2  "<dot_d_analytical_mps>"
  Bus Selector5/2 -> Bus Creator/3  "<dot_d_numerical_mps>"

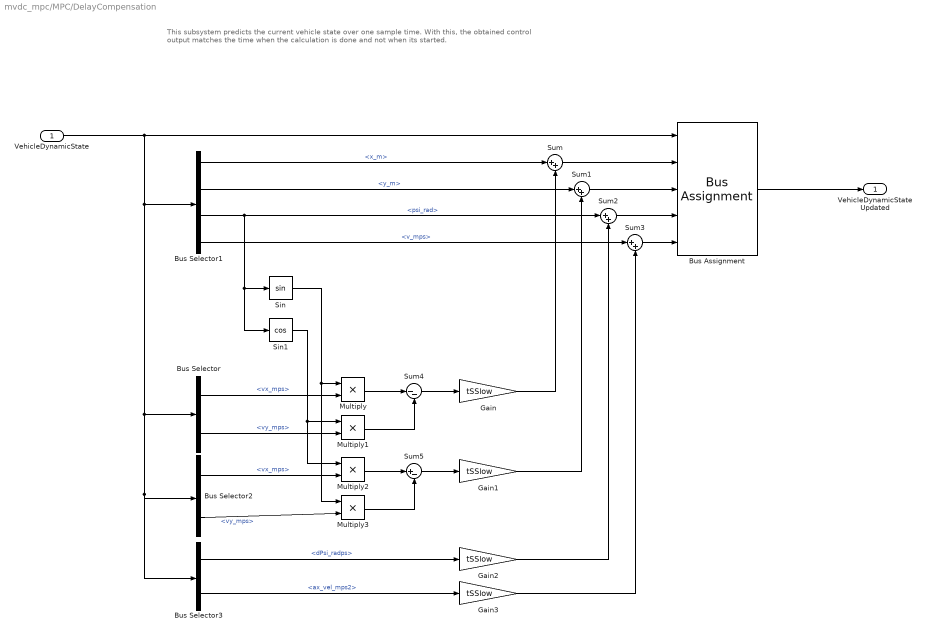
== system mvdc_mpc/MPC/DelayCompensation ==
  note: This subsystem predicts the current vehicle state over one sample time.
      | With this, the obtained control output matches the time when the calculation is done and not when its started.
  VehicleDynamicState : Inport
  Bus Assignment : BusAssignment  AssignedSignals=Pos.x_m,Pos.y_m,Pos.psi_rad,v_mps
  Bus Selector : BusSelector  OutputSignals=vx_mps,vy_mps
  Bus Selector1 : BusSelector  OutputSignals=Pos.x_m,Pos.y_m,Pos.psi_rad,v_mps
  Bus Selector2 : BusSelector  OutputSignals=vx_mps,vy_mps
  Bus Selector3 : BusSelector  OutputSignals=dPsi_radps,ax_vel_mps2
  Gain{,1..3} (4 alike) : Gain  Gain=tSSlow
  Multiply{,1..3} (4 alike) : Product
  Sin : Trigonometry
  Sin1 : Trigonometry  Operator=cos
  Sum{,1..3} (4 alike) : Sum  Inputs=|++
  Sum4 : Sum  Inputs=|--
  Sum5 : Sum  Inputs=|+-
  VehicleDynamicStateUpdated : Outport
  wires:
  Bus Assignment/1 -> VehicleDynamicStateUpdated/1
  Bus Selector1/1 -> Sum/1  "<x_m>"
  Sum/1 -> Bus Assignment/2
  Bus Selector1/2 -> Sum1/1  "<y_m>"
  Sum1/1 -> Bus Assignment/3
  Bus Selector1/3 -> Sin1/1, Sin/1, Sum2/1  "<psi_rad>"
  Sum2/1 -> Bus Assignment/4
  Sum3/1 -> Bus Assignment/5
  Bus Selector1/4 -> Sum3/1  "<v_mps>"
  Bus Selector/1 -> Multiply/2  "<vx_mps>"
  Sin/1 -> Multiply3/1, Multiply/1
  Bus Selector/2 -> Multiply1/2  "<vy_mps>"
  Sin1/1 -> Multiply2/1, Multiply1/1
  Multiply/1 -> Sum4/1
  Multiply1/1 -> Sum4/2
  Sum4/1 -> Gain/1
  Gain/1 -> Sum/2
  VehicleDynamicState/1 -> Bus Selector3/1, Bus Selector2/1, Bus Selector/1, Bus Selector1/1, Bus Assignment/1
  Bus Selector2/1 -> Multiply2/2  "<vx_mps>"
  Bus Selector2/2 -> Multiply3/2  "<vy_mps>"
  Multiply2/1 -> Sum5/1
  Multiply3/1 -> Sum5/2
  Sum5/1 -> Gain1/1
  Gain1/1 -> Sum1/2
  Bus Selector3/1 -> Gain2/1  "<dPsi_radps>"
  Bus Selector3/2 -> Gain3/1  "<ax_vel_mps2>"
  Gain2/1 -> Sum2/2
  Gain3/1 -> Sum3/2

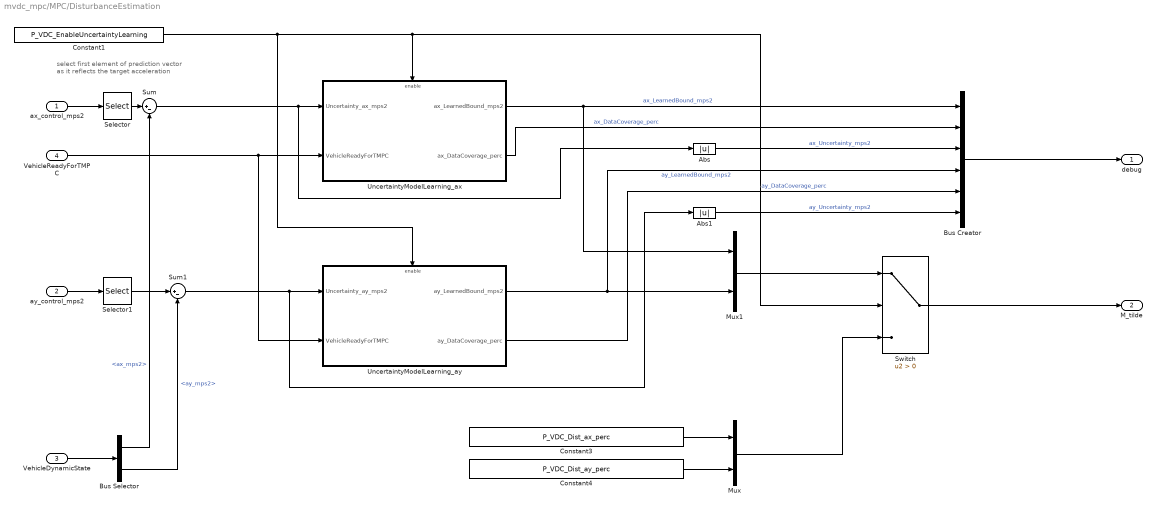
== system mvdc_mpc/MPC/DisturbanceEstimation ==
  note: select first element of prediction vector
      | as it reflects the target acceleration
  ax_control_mps2 : Inport
  ay_control_mps2 : Inport  Port=2
  VehicleDynamicState : Inport  Port=3
  VehicleReadyForTMPC : Inport  Port=4
  Abs : Abs
  Abs1 : Abs
  Bus Creator : BusCreator  Inputs=6
  Bus Selector : BusSelector  OutputSignals=ax_mps2,ay_mps2
  Constant1 : Constant  Value=P_VDC_EnableUncertaintyLearning
  Constant3 : Constant  Value=P_VDC_Dist_ax_perc
  Constant4 : Constant  Value=P_VDC_Dist_ay_perc
  Mux : Mux  Inputs=2
  Mux1 : Mux  Inputs=2
  Selector : Selector  InputPortWidth=sys.N_hor+1  IndexOptions=Index vector (dialog)  Indices=[1]  OutputSizes=1
  Selector1 : Selector  InputPortWidth=sys.N_hor+1  IndexOptions=Index vector (dialog)  Indices=[1]  OutputSizes=1
  Sum : Sum  Inputs=|+-
  Sum1 : Sum  Inputs=|+-
  Switch : Switch  Criteria=u2 > Threshold
  UncertaintyModelLearning_ax : Subsystem
  UncertaintyModelLearning_ay : Subsystem
  debug : Outport
  M_tilde : Outport  Port=2
  wires:
  VehicleDynamicState/1 -> Bus Selector/1
  ax_control_mps2/1 -> Selector/1
  Bus Selector/2 -> Sum1/2  "<ay_mps2>"
  Bus Selector/1 -> Sum/2  "<ax_mps2>"
  Sum/1 -> Abs/1, UncertaintyModelLearning_ax/1(Uncertainty_ax_mps2)
  Constant4/1 -> Mux/2
  Constant3/1 -> Mux/1
  ay_control_mps2/1 -> Selector1/1
  Sum1/1 -> UncertaintyModelLearning_ay/1(Uncertainty_ay_mps2), Abs1/1
  Mux/1 -> Switch/3
  UncertaintyModelLearning_ay/1(ay_LearnedBound_mps2) -> Bus Creator/4, Mux1/2  "ay_LearnedBound_mps2"
  Mux1/1 -> Switch/1
  Constant1/1 -> UncertaintyModelLearning_ay/Enable, UncertaintyModelLearning_ax/Enable, Switch/2
  Bus Creator/1 -> debug/1
  UncertaintyModelLearning_ax/1(ax_LearnedBound_mps2) -> Mux1/1, Bus Creator/1  "ax_LearnedBound_mps2"
  UncertaintyModelLearning_ax/2(ax_DataCoverage_perc) -> Bus Creator/2  "ax_DataCoverage_perc"
  UncertaintyModelLearning_ay/2(ay_DataCoverage_perc) -> Bus Creator/5  "ay_DataCoverage_perc"
  Abs/1 -> Bus Creator/3  "ax_Uncertainty_mps2"
  Abs1/1 -> Bus Creator/6  "ay_Uncertainty_mps2"
  VehicleReadyForTMPC/1 -> UncertaintyModelLearning_ay/2(VehicleReadyForTMPC), UncertaintyModelLearning_ax/2(VehicleReadyForTMPC)
  Selector/1 -> Sum/1
  Selector1/1 -> Sum1/1
  Switch/1 -> M_tilde/1

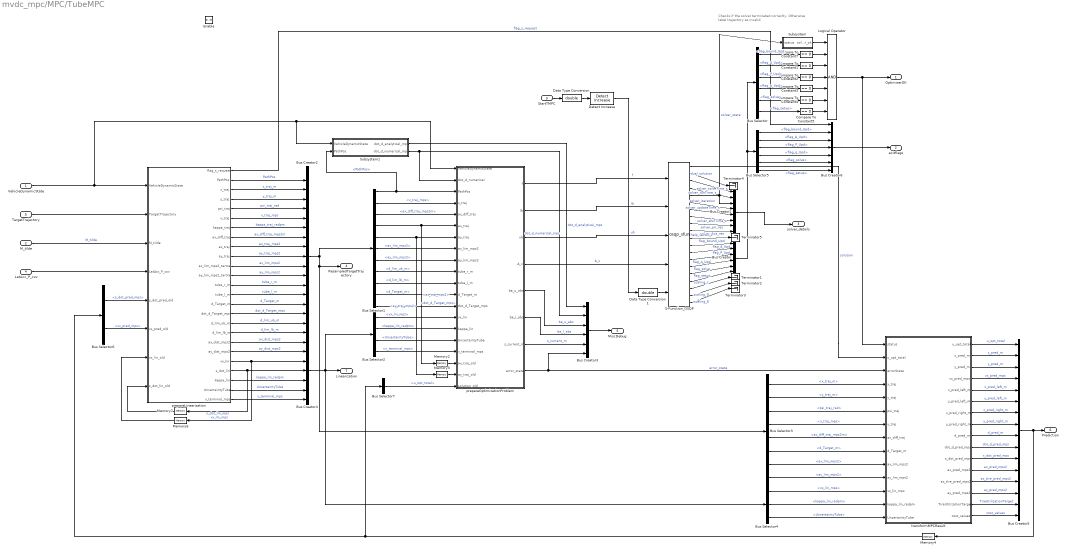
== system mvdc_mpc/MPC/TubeMPC ==
  note: Checks if the solver terminated correctly. Otherwise
      | label trajectory as invalid.
  VehicleDynamicState : Inport
  M_tilde : Inport  Port=2
  StartTMPC : Inport  Port=3  OutDataTypeStr=boolean  SampleTime=tS
  LatAcc_P_cov : Inport  Port=4
  TargetTrajectory : Inport  Port=5
  Enable : EnablePort
  Bus Creator : BusCreator  Inputs=6
  Bus Creator1 : BusCreator  Inputs=8
  Bus Creator2 : BusCreator  Inputs=17
  Bus Creator3 : BusCreator  Inputs=6
  Bus Creator4 : BusCreator  Inputs=7
  Bus Creator5 : BusCreator  Inputs=16
  Bus Creator6 : BusCreator  Inputs=7
  Bus Selector : BusSelector  OutputSignals=flag_bound_Upd,flag_A_Upd,flag_P_Upd,flag_q_Upd,flag_solve,flag_setup
  Bus Selector1 : BusSelector  OutputSignals=PathPos,v_traj_mps,ax_diff_traj_mps2m,ax_traj_mps2,ay_traj_mps2,ax_lim_mps2,ay_lim_mps2,d_lim_ub_m,d_lim_lb_m,d_Target_m,dot_d_Target_mps
  Bus Selector2 : BusSelector  OutputSignals=vx_lin_mps,kappa_lin_radpm,UncertaintyTube,v_terminal_mps
  Bus Selector3 : BusSelector  OutputSignals=x_traj_m,y_traj_m,psi_traj_rad,v_traj_mps,ax_diff_traj_mps2m,d_Target_m,ax_lim_mps2,ay_lim_mps2
  Bus Selector4 : BusSelector  OutputSignals=vx_lin_mps,kappa_lin_radpm,UncertaintyTube
  Bus Selector5 : BusSelector  OutputSignals=flag_bound_Upd,flag_A_Upd,flag_P_Upd,flag_q_Upd,flag_solve,flag_setup
  Bus Selector6 : BusSelector  OutputSignals=s_dot_pred_mps,vx_pred_mps
  Bus Selector7 : BusSelector  OutputSignals=u_opt_total
  Compare To Constant{1..5,7} (6 alike) : simulink/Logic and Bit Operations/Compare To Constant  relop===  const=0  OutDataTypeStr=boolean
  Data Type Conversion : DataTypeConversion  OutDataTypeStr=double
  Data Type Conversion1 : DataTypeConversion  OutDataTypeStr=double
  Detect Increase : simulink/Logic and Bit Operations/Detect Increase  vinit=0.0  OutDataTypeStr=boolean
  Logical Operator : Logic  Inputs=7  AllPortsSameDT=off  OutDataTypeStr=boolean
  Memory{2..4,6..7} (5 alike) : Memory  InheritSampleTime=on
  S-Function_OSQP : S-Function  FunctionName=osqp_sfun  Parameters=sys.osqp_qpar', sys.osqp_m, sys.osqp_n, sys.P_x_par, sys.P_i_par, sys.P_p_par, sys.A_x_par, sys.A_i_par, sys.A_p_par, sys.l_par', sys.u_par', sys.trigger_print, P_VDC_TMPCMaxSolverIter  SFunctionDeploymentMode=off  EnableBusSupport=off
  Subsystem : Subsystem
  Subsystem1 : Subsystem
  Terminator{1..5} (5 alike) : Terminator
  prepareLinearization : MATLAB Function  TreatAsAtomicUnit=on
  prepareOptimizationProblem : MATLAB Function  TreatAsAtomicUnit=on
  transformMPCResult : MATLAB Function  TreatAsAtomicUnit=on
  OptimizerOK : Outport  OutDataTypeStr=boolean
  exitflags : Outport  Port=2
  solver_details : Outport  Port=3
  ResampledTargetTrajectory : Outport  Port=4
  MiscDebug : Outport  Port=5
  Prediction : Outport  Port=6
  Linearization : Outport  Port=7
  wires:
  prepareLinearization/3(x_traj) -> Bus Creator2/2  "x_traj_m"
  transformMPCResult/4(vx_pred_mps) -> Bus Creator5/4  "vx_pred_mps"
  prepareLinearization/6(v_traj) -> Bus Creator2/5  "v_traj_mps"
  prepareOptimizationProblem/8(error_state) -> Bus Creator3/6, transformMPCResult/3(errorState)  "error_state"
  prepareLinearization/7(kappa_traj) -> Bus Creator2/6  "kappa_traj_radpm"
  prepareLinearization/4(y_traj) -> Bus Creator2/3  "y_traj_m"
  prepareLinearization/5(psi_traj) -> Bus Creator2/4  "psi_traj_rad"
  TargetTrajectory/1 -> prepareLinearization/2(TargetTrajectory)
  prepareOptimizationProblem/2(lb) -> S-Function_OSQP/2  "lb"
  prepareOptimizationProblem/4(A_x) -> S-Function_OSQP/4  "A_x"
  prepareOptimizationProblem/1(f) -> S-Function_OSQP/1  "f"
  S-Function_OSQP/5 -> Bus Creator1/3, Subsystem/1(status)  "solver_state"
  prepareOptimizationProblem/3(ub) -> S-Function_OSQP/3  "ub"
  S-Function_OSQP/12 -> Bus Creator/1  "flag_bound_Upd"
  S-Function_OSQP/13 -> Bus Creator/2  "flag_A_Upd"
  S-Function_OSQP/14 -> Bus Creator/3  "flag_P_Upd"
  S-Function_OSQP/15 -> Bus Creator/4  "flag_q_Upd"
  S-Function_OSQP/16 -> Bus Creator/5  "flag_solve"
  S-Function_OSQP/17 -> Bus Creator/6  "flag_setup"
  S-Function_OSQP/3 -> Bus Creator1/1  "solver_solveTime_s"
  S-Function_OSQP/4 -> Bus Creator1/2  "solver_runTime_s"
  S-Function_OSQP/8 -> Bus Creator1/6  "solver_sfunTime_s"
  S-Function_OSQP/7 -> Bus Creator1/5  "solver_updateTime_s"
  S-Function_OSQP/6 -> Bus Creator1/4  "solver_iteration"
  Bus Creator1/1 -> solver_details/1
  Bus Creator3/1 -> MiscDebug/1
  Logical Operator/1 -> OptimizerOK/1, transformMPCResult/1(status)
  prepareLinearization/1(flag_s_request) -> Bus Creator6/1  "flag_s_request"
  Compare To Constant5/1 -> Logical Operator/7
  Compare To Constant4/1 -> Logical Operator/6
  Compare To Constant3/1 -> Logical Operator/5
  Compare To Constant2/1 -> Logical Operator/4
  Compare To Constant1/1 -> Logical Operator/3
  Compare To Constant7/1 -> Logical Operator/2
  Bus Creator4/1 -> Bus Selector2/1, Linearization/1, Bus Selector4/1
  S-Function_OSQP/18 -> Terminator1/1  "scaling_c"
  S-Function_OSQP/19 -> Terminator2/1  "scaling_D"
  S-Function_OSQP/20 -> Terminator3/1  "scaling_E"
  S-Function_OSQP/9 -> Bus Creator1/7  "solver_pri_res"
  S-Function_OSQP/10 -> Bus Creator1/8  "solver_dua_res"
  transformMPCResult/14(ay_pred_mps2) -> Bus Creator5/14  "ay_pred_mps2"
  S-Function_OSQP/1 -> transformMPCResult/2("u_opt_total ")  "solution"
  Subsystem/1(solver_ok) -> Logical Operator/1
  prepareOptimizationProblem/6(be_l_abs) -> Bus Creator3/4  "be_l_abs"
  prepareOptimizationProblem/5(be_u_abs) -> Bus Creator3/3  "be_u_abs"
  transformMPCResult/1(u_opt_total) -> Bus Creator5/1  "u_opt_total"
  transformMPCResult/2(x_pred_m) -> Bus Creator5/2  "x_pred_m"
  transformMPCResult/3(y_pred_m) -> Bus Creator5/3  "y_pred_m"
  transformMPCResult/10(dot_d_pred_mps) -> Bus Creator5/10  "dot_d_pred_mps"
  transformMPCResult/9(d_pred_m) -> Bus Creator5/9  "d_pred_m"
  transformMPCResult/11(s_dot_pred_mps) -> Bus Creator5/11  "s_dot_pred_mps"
  prepareLinearization/8(ax_diff_traj) -> Bus Creator2/7  "ax_diff_traj_mps2m"
  prepareLinearization/21(vx_lin) -> Memory6/1, Bus Creator4/3  "vx_lin_mps"
  prepareLinearization/22(s_dot_lin) -> Memory7/1, Bus Creator4/4  "s_dot_lin_mps"
  prepareLinearization/9(ax_traj) -> Bus Creator2/8  "ax_traj_mps2"
  prepareLinearization/10(ay_traj) -> Bus Creator2/9  "ay_traj_mps2"
  transformMPCResult/13(ax_tire_pred_mps2) -> Bus Creator5/13  "ax_tire_pred_mps2"
  prepareLinearization/17(d_lim_ub_m) -> Bus Creator2/16  "d_lim_ub_m"
  prepareLinearization/12(ay_lim_mps2_tartraj) -> Bus Creator2/11  "ay_lim_mps2"
  prepareLinearization/11(ax_lim_mps2_tartraj) -> Bus Creator2/10  "ax_lim_mps2"
  prepareLinearization/15(d_Target_m) -> Bus Creator2/14  "d_Target_m"
  prepareLinearization/16(dot_d_Target_mps) -> Bus Creator2/15  "dot_d_Target_mps"
  prepareLinearization/18(d_lim_lb_m) -> Bus Creator2/17  "d_lim_lb_m"
  Memory6/1 -> prepareLinearization/7(vx_lin_old)
  Memory7/1 -> prepareLinearization/8(s_dot_lin_old)
  prepareLinearization/23(kappa_lin) -> Bus Creator4/5  "kappa_lin_radpm"
  transformMPCResult/12(ax_pred_mps2) -> Bus Creator5/12  "ax_pred_mps2"
  S-Function_OSQP/2 -> Terminator4/1  "dual_solution"
  S-Function_OSQP/11 -> Terminator5/1  "help_vector_z"
  transformMPCResult/8(y_pred_right_m) -> Bus Creator5/8  "y_pred_right_m"
  transformMPCResult/7(x_pred_right_m) -> Bus Creator5/7  "x_pred_right_m"
  transformMPCResult/6(y_pred_left_m) -> Bus Creator5/6  "y_pred_left_m"
  transformMPCResult/5(x_pred_left_m) -> Bus Creator5/5  "x_pred_left_m"
  Bus Creator5/1 -> Memory4/1, Prediction/1
  prepareLinearization/20(ay_dist_mps2) -> Bus Creator4/2  "ay_dist_mps2"
  prepareLinearization/19(ax_dist_mps2) -> Bus Creator4/1  "ax_dist_mps2"
  M_tilde/1 -> prepareLinearization/3(M_tilde)  "M_tilde"
  prepareLinearization/13(tube_r_m) -> Bus Creator2/12  "tube_r_m"
  prepareLinearization/14(tube_l_m) -> Bus Creator2/13  "tube_l_m"
  Bus Creator/1 -> Bus Selector/1, Bus Selector5/1
  Bus Selector/1 -> Compare To Constant7/1  "<flag_bound_Upd>"
  Bus Selector/2 -> Compare To Constant1/1  "<flag_A_Upd>"
  Bus Selector/3 -> Compare To Constant2/1  "<flag_P_Upd>"
  Bus Selector/4 -> Compare To Constant3/1  "<flag_q_Upd>"
  Bus Selector/5 -> Compare To Constant4/1  "<flag_solve>"
  Bus Selector/6 -> Compare To Constant5/1  "<flag_setup>"
  Bus Creator2/1 -> Bus Selector3/1, ResampledTargetTrajectory/1, Bus Selector1/1
  Bus Selector1/2 -> prepareOptimizationProblem/4(v_traj)  "<v_traj_mps>"
  Bus Selector1/3 -> prepareOptimizationProblem/5(ax_diff_traj)  "<ax_diff_traj_mps2m>"
  Bus Selector1/4 -> Memory2/1, prepareOptimizationProblem/6(ax_traj)  "<ax_traj_mps2>"
  Bus Selector1/5 -> Memory3/1, prepareOptimizationProblem/7(ay_traj)  "<ay_traj_mps2>"
  Bus Selector1/6 -> prepareOptimizationProblem/8(ax_lim_mps2)  "<ax_lim_mps2>"
  Bus Selector1/7 -> prepareOptimizationProblem/9(ay_lim_mps2)  "<ay_lim_mps2>"
  Bus Selector1/8 -> prepareOptimizationProblem/10(tube_r_m)  "<d_lim_ub_m>"
  Bus Selector1/9 -> prepareOptimizationProblem/11(tube_l_m)  "<d_lim_lb_m>"
  Bus Selector1/10 -> prepareOptimizationProblem/12(d_Target_m)  "<d_Target_m>"
  Bus Selector1/11 -> prepareOptimizationProblem/13(dot_d_Target_mps)  "<dot_d_Target_mps>"
  Bus Selector2/2 -> prepareOptimizationProblem/15(kappa_lin)  "<kappa_lin_radpm>"
  Bus Selector2/1 -> prepareOptimizationProblem/14(vx_lin)  "<vx_lin_mps>"
  transformMPCResult/15(TireUtilizationTarget) -> Bus Creator5/15  "TireUtilizationTarget"
  transformMPCResult/16(cost_values) -> Bus Creator5/16  "cost_values"
  Memory2/1 -> prepareOptimizationProblem/18(ax_traj_old)
  Memory3/1 -> prepareOptimizationProblem/19(ay_traj_old)
  Bus Selector3/1 -> transformMPCResult/4(x_traj)  "<x_traj_m>"
  Bus Selector3/2 -> transformMPCResult/5(y_traj)  "<y_traj_m>"
  Bus Selector3/3 -> transformMPCResult/6(psi_traj)  "<psi_traj_rad>"
  Bus Selector3/4 -> transformMPCResult/7(v_traj)  "<v_traj_mps>"
  Bus Selector3/5 -> transformMPCResult/8(ax_diff_traj)  "<ax_diff_traj_mps2m>"
  Bus Selector3/6 -> transformMPCResult/9(d_Target_m)  "<d_Target_m>"
  Bus Selector3/7 -> transformMPCResult/10(ax_lim_mps2)  "<ax_lim_mps2>"
  Bus Selector3/8 -> transformMPCResult/11(ay_lim_mps2)  "<ay_lim_mps2>"
  Bus Selector4/1 -> transformMPCResult/12(vx_lin_mps)  "<vx_lin_mps>"
  Bus Selector4/2 -> transformMPCResult/13(kappa_lin_radpm)  "<kappa_lin_radpm>"
  Bus Selector5/1 -> Bus Creator6/2  "<flag_bound_Upd>"
  Bus Selector5/2 -> Bus Creator6/3  "<flag_A_Upd>"
  Bus Selector5/3 -> Bus Creator6/4  "<flag_P_Upd>"
  Bus Selector5/4 -> Bus Creator6/5  "<flag_q_Upd>"
  Bus Selector5/5 -> Bus Creator6/6  "<flag_solve>"
  Bus Selector5/6 -> Bus Creator6/7  "<flag_setup>"
  Bus Creator6/1 -> exitflags/1
  Memory4/1 -> Bus Selector7/1, Bus Selector6/1
  Bus Selector6/1 -> prepareLinearization/5(s_dot_pred_old)  "<s_dot_pred_mps>"
  Bus Selector6/2 -> prepareLinearization/6(vx_pred_old)  "<vx_pred_mps>"
  Bus Selector7/1 -> prepareOptimizationProblem/20(solution_old)  "<u_opt_total>"
  prepareLinearization/24(UncertaintyTube) -> Bus Creator4/6  "UncertaintyTube"
  Bus Selector4/3 -> transformMPCResult/14(UncertaintyTube)  "<UncertaintyTube>"
  Bus Selector2/3 -> prepareOptimizationProblem/16(UncertaintyTube)  "<UncertaintyTube>"
  prepareOptimizationProblem/7(s_current_m) -> Bus Creator3/5  "s_current_m"
  prepareLinearization/2(PathPos) -> Bus Creator2/1  "PathPos"
  Bus Selector1/1 -> Subsystem1/2(PathPos), prepareOptimizationProblem/3(PathPos)  "<PathPos>"
  LatAcc_P_cov/1 -> prepareLinearization/4(LatAcc_P_cov)
  prepareLinearization/25(v_terminal_mps) -> Bus Creator4/7  "v_terminal_mps"
  Bus Selector2/4 -> prepareOptimizationProblem/17(v_terminal_mps)  "<v_terminal_mps>"
  StartTMPC/1 -> Data Type Conversion/1
  Data Type Conversion/1 -> Detect Increase/1
  Detect Increase/1 -> Data Type Conversion1/1
  Data Type Conversion1/1 -> S-Function_OSQP/5
  Subsystem1/2(dot_d_numerical_mps) -> Bus Creator3/2, prepareOptimizationProblem/2(dot_d_numerical)  "dot_d_numerical_mps"
  VehicleDynamicState/1 -> Subsystem1/1(VehicleDynamicState), prepareOptimizationProblem/1(VehicleDynamicState), prepareLinearization/1(VehicleDynamicState)
  Subsystem1/1(dot_d_analytical_mps) -> Bus Creator3/1  "dot_d_analytical_mps"

== system mvdc_mpc/MPC/VehicleReadyForTMPC ==
  note: TMPC calculations are allowed once
      | 	- The state estimation is valid
      | 	- The target trajectory is valid
  VehicleDynamicState : Inport
  TargetTrajectory : Inport  Port=2
  EnableDrivingController : Inport  Port=3  OutDataTypeStr=boolean  SampleTime=tS
  Bus Selector2 : BusSelector  OutputSignals=SE_Status
  Bus Selector3 : BusSelector  OutputSignals=TrajCnt
  Compare To Constant1 : simulink/Logic and Bit Operations/Compare To Constant  relop=>=  const=TUMHealthStatus.WARNING  OutDataTypeStr=boolean
  Compare To Constant2 : simulink/Logic and Bit Operations/Compare To Constant  relop=>=  const=1  OutDataTypeStr=boolean
  Constant : Constant  Value=P_VDC_EnableTubeMPC
  Logical Operator : Logic  Inputs=3  AllPortsSameDT=off  OutDataTypeStr=boolean
  Logical Operator1 : Logic  AllPortsSameDT=off  OutDataTypeStr=boolean
  VehicleReadyForTMPC : Outport
  StartTMPC : Outport  Port=2
  wires:
  Bus Selector3/1 -> Compare To Constant2/1  "<TrajCnt>"
  VehicleDynamicState/1 -> Bus Selector2/1
  Logical Operator/1 -> Logical Operator1/1, VehicleReadyForTMPC/1
  TargetTrajectory/1 -> Bus Selector3/1
  Bus Selector2/1 -> Compare To Constant1/1  "<SE_Status>"
  Compare To Constant2/1 -> Logical Operator/3
  Compare To Constant1/1 -> Logical Operator/2
  Constant/1 -> Logical Operator/1
  EnableDrivingController/1 -> Logical Operator1/2
  Logical Operator1/1 -> StartTMPC/1
